simulink model "GeneralDynamics"  (R2025a)
settings: Solver=VariableStepAuto  StartTime=0.0  StopTime=10.0  RelTol=1e-3
libraries: aerolibanim x1
settings Model: Creator=sh2323  LastModifiedBy=sh2323

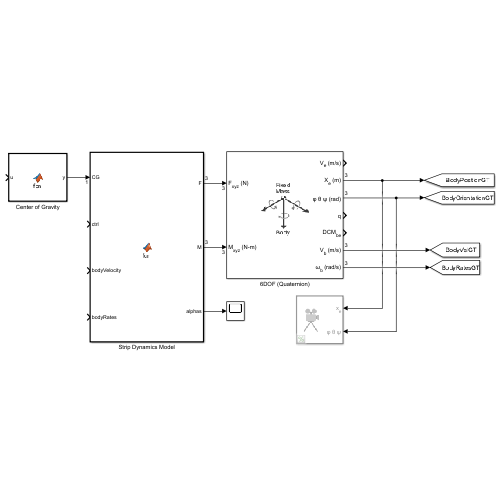
[thumbnail: Simulink's stored preview of the top-level diagram]
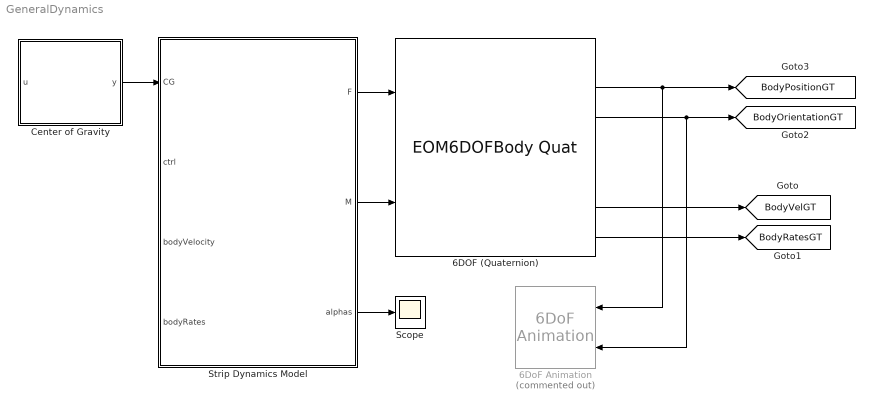
== system GeneralDynamics ==
  6DOF (Quaternion) : EOM6DOFBodyQuat
  6DoF Animation : aerolibanim/6DoF Animation  Commented=on  u1=[0 4000 -2000 2000 -5000 -3000]  u2=0.1  u3=1.0  u4=[4000 0 -5000]  u5=Fixed position  u6=[2000 500 -3150]  u7=10  u8=on
  Center of Gravity : MATLAB Function  TreatAsAtomicUnit=on
  Scope : Scope
  Strip Dynamics Model : MATLAB Function  TreatAsAtomicUnit=on
  tag scope: BodyOrientationGT=global, BodyPositionGT=global, BodyRatesGT=global, BodyVelGT=global
  wires:
  Strip Dynamics Model/1(F) -> 6DOF (Quaternion)/1
  Strip Dynamics Model/2(M) -> 6DOF (Quaternion)/2
  Strip Dynamics Model/3(alphas) -> Scope/1
  6DOF (Quaternion)/2 -> [BodyPositionGT], 6DoF Animation/1
  6DOF (Quaternion)/3 -> [BodyOrientationGT], 6DoF Animation/2
  6DOF (Quaternion)/6 -> [BodyVelGT]
  6DOF (Quaternion)/7 -> [BodyRatesGT]
  Center of Gravity/1(y) -> Strip Dynamics Model/1(CG)

== matlab function GeneralDynamics/Center of Gravity ==
  data: u input; y output
function y = fcn(u)

y = u;

== matlab function GeneralDynamics/Strip Dynamics Model ==
  data: CG input; ctrl input; bodyVelocity input; bodyRates input; F output; M output; alphas output
function [F,M,alphas] = fcn(CG,ctrl,bodyVelocity,bodyRates)

y = u;
